simulink model "tmu_ref_am13x"  (R2025b)
settings: Solver=FixedStepAuto  StartTime=0.0  StopTime=1  RelTol=1e-3  EnableMultiTasking=on
settings Model: SimulationMode=processor-in-the-loop (pil)  CodeVerificationMode=processor-in-the-loop (pil)  Creator=a1255762  LastModifiedBy=a1255762
settings OptimizationCC: DefaultUnderspecifiedDataType=single  EnhancedBackFolding=on  PassReuseOutputArgsAs=Individual arguments  ZeroExternalMemoryAtStartup=off  ZeroInternalMemoryAtStartup=off  MaxStackSize=64  OptimizeBlockOrder=speed  DifferentSizesBufferReuse=on  OptimizationCustomize=off  EfficientTunableParamExpr=on
settings DebuggingCC: ParameterPrecisionLossMsg=none  ParameterTunabilityLossMsg=error
settings HardwareCC: ProdBitPerPointer=32.0  ProdBitPerSizeT=32.0  ProdBitPerPtrDiffT=32.0  ProdLargestAtomicInteger=Long  ProdLargestAtomicFloat=Double  ProdWordSize=32.0  ProdLongLongMode=on  ProdHWDeviceType=ARM Compatible->ARM Cortex
settings SFSimCC: MATLABDynamicMemAlloc=off
settings RTWCC: SystemTargetFile=ert.tlc  HardwareBoard=AM13E230x  TemplateMakefile=ert_default_tmf  GenerateReport=on  Toolchain=TI ARM Clang Compiler AM13x | gmake  BuildConfiguration=Faster Runs  IncludeHyperlinkInReport=on  LaunchReport=on  CodeExecutionProfiling=on  CodeProfilingInstrumentation=detailed  GenerateTraceInfo=on  GenerateCodeReplacementReport=on  Description=Embedded Coder
settings CodeAppCC: ForceParamTrailComments=on  IgnoreCustomStorageClasses=off  MaxIdLength=256.0  OperatorAnnotations=on  SimulinkDataObjDesc=on  SFDataObjDesc=on  InsertBlockDesc=on
settings ERTTargetCC: ExtModeTransport=3.0  ExtModeStaticAlloc=on  ExtModeMexFile=ext_xcp  ExtModeIntrfLevel=Level2 - Open  InlinedParameterPlacement=Hierarchical  ERTCustomFileTemplate=AM13x_codertarget_file_process.tlc  CodeReplacementLibrary=AM13x_TMU

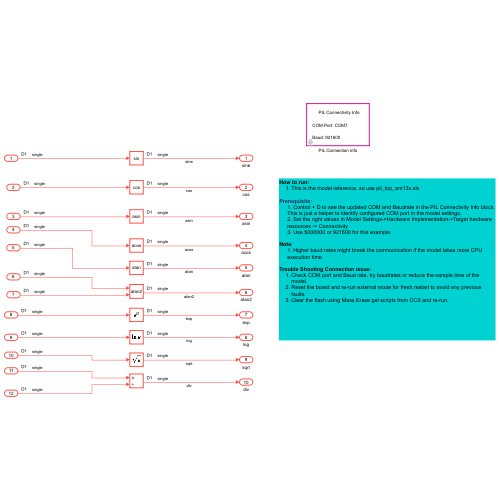
[thumbnail: Simulink's stored preview of the top-level diagram]
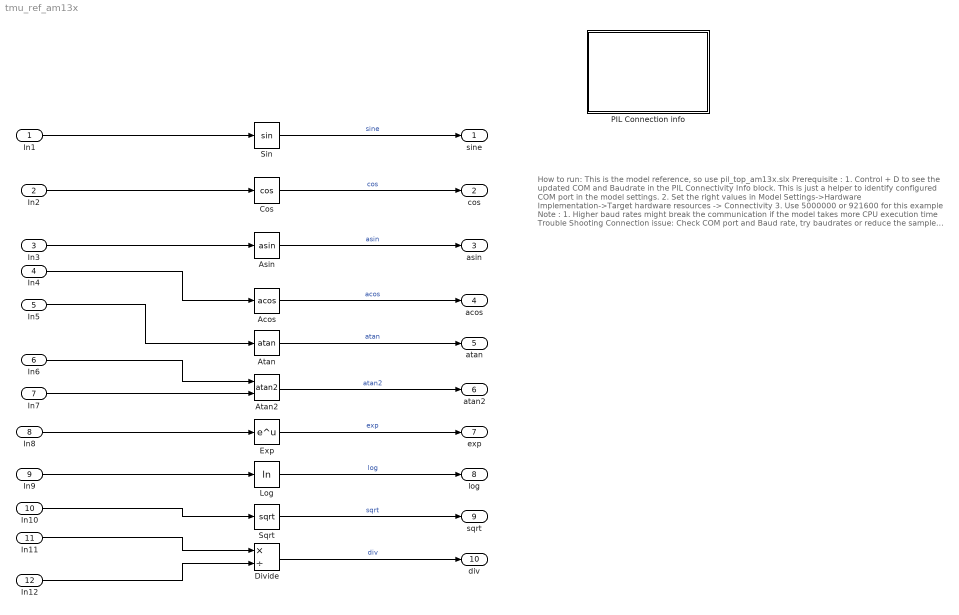
== system tmu_ref_am13x ==
  note: How to run:
      | This is the model reference, so use pil_top_am13x.slx
      |
      | Prerequisite :
      | 1. Control + D to see the updated COM and Baudrate in the PIL Connectivity Info block. This is just a helper to identify configured COM port in the model settings.
      | 2. Set the right values in Model Settings->Hardware Implementation->Target hardware resources -> Connectivity
      | 3. Use 5000000 or 921600 for this example
      |
      | Note :
      | 1. Higher baud rates might break the communication if the model takes more CPU execution time
      |
      | Trouble Shooting Connection issue:
      | Check COM port and Baud rate, try baudrates or reduce the sample time of the model.
      | Reset the board and re-run external mode for fresh restart to avoid any previous faults.
      | Clear the flash using Mass Erase gel scripts from CCS and re-run.
  In1 : Inport
  In2 : Inport  Port=2
  In3 : Inport  Port=3
  In4 : Inport  Port=4
  In5 : Inport  Port=5
  In6 : Inport  Port=6
  In7 : Inport  Port=7
  In8 : Inport  Port=8
  In9 : Inport  Port=9
  In10 : Inport  Port=10
  In11 : Inport  Port=11
  In12 : Inport  Port=12
  Acos : Trigonometry  Operator=acos
  Asin : Trigonometry  Operator=asin
  Atan : Trigonometry  Operator=atan
  Atan2 : Trigonometry  Operator=atan2
  Cos : Trigonometry  Operator=cos
  Divide : Product  Inputs=*/  OutDataTypeStr=single
  Exp : Math
  Log : Math  Operator=log
  PIL Connection info : Subsystem  mask{Parameter1=|}
      mask Parameter1=|
      | codertarget.data.setParameterValue(bdroot, 'Connection.Serialport', 'COM3')
      | codertarget.data.setParameterValue(bdroot, 'Connection.Baud', '5000000')
      mask prompts: Parameter1 "Change programmatically"
      mask Display:
      | % Update mask parameters with current values when opened
      | 
      | pilData = codertarget.data.getParameterValue(bdroot, 'Connection');
      | 
      | 
      | % Use text() function with specific positioning
      | text(0.2, 0.8, 'PIL Connectivity Info', 'HorizontalAlignment', 'left');
      | text(0.1, 0.5, ['COM Port: ' pilData.Serialport], 'HorizontalAlignment', 'left');
      | text(0.1, 0.2, ['Baud: ' pilData.Baud], 'HorizontalAlignment', 'left');
  Sin : Trigonometry
  Sqrt : Sqrt
  sine : Outport
  cos : Outport  Port=2
  asin : Outport  Port=3
  acos : Outport  Port=4
  atan : Outport  Port=5
  atan2 : Outport  Port=6
  exp : Outport  Port=7
  log : Outport  Port=8
  sqrt : Outport  Port=9
  div : Outport  Port=10
  wires:
  Atan/1 -> atan/1  "atan"
  In6/1 -> Atan2/1
  In4/1 -> Acos/1
  In3/1 -> Asin/1
  In9/1 -> Log/1
  Cos/1 -> cos/1  "cos"
  Acos/1 -> acos/1  "acos"
  Asin/1 -> asin/1  "asin"
  Sqrt/1 -> sqrt/1  "sqrt"
  In10/1 -> Sqrt/1
  In7/1 -> Atan2/2
  Exp/1 -> exp/1  "exp"
  Log/1 -> log/1  "log"
  Atan2/1 -> atan2/1  "atan2"
  In8/1 -> Exp/1
  Divide/1 -> div/1  "div"
  In2/1 -> Cos/1
  In5/1 -> Atan/1
  In11/1 -> Divide/1
  In1/1 -> Sin/1
  Sin/1 -> sine/1  "sine"
  In12/1 -> Divide/2

== system tmu_ref_am13x/PIL Connection info ==
